simulink model "DPT_Posl_Podkl"  (R2023a)
settings: Solver=VariableStepAuto  StartTime=0.0  StopTime=10.0  RelTol=1e-3
values from neighbouring files (symbols this model uses):
  beta = 0.001    [Constants.m]
  C_m = 1.3    [Constants.m]
  C_w = 3.15    [Constants.m]
  J_dv = 7 * 10^(-6)    (= 7e-06)    [Constants.m]
  L_a = 0.0015    [Constants.m]
  L_ov = 0.013    [Constants.m]
  R_a = 8    [Constants.m]
settings Model: Creator=George  LastModifiedBy=George

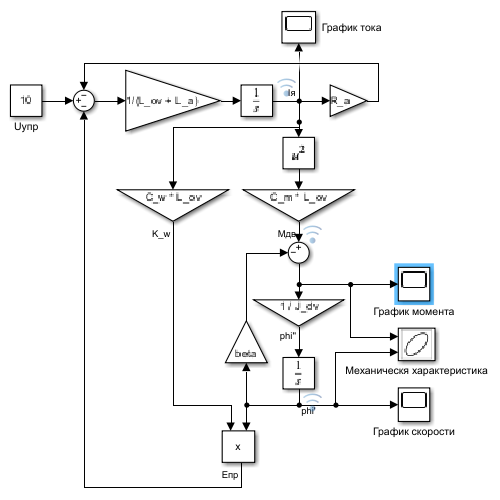
[thumbnail: Simulink's stored preview of the top-level diagram]
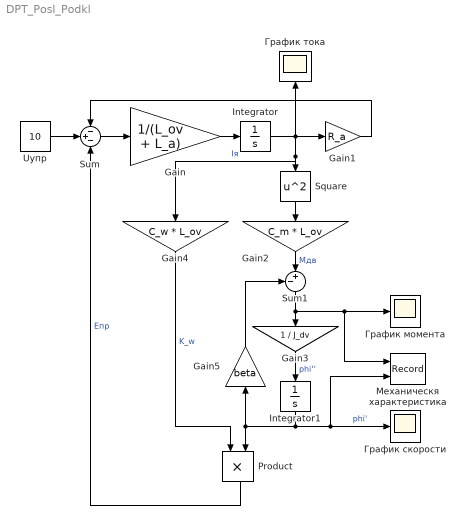
== system DPT_Posl_Podkl ==
  Gain : Gain  Gain=1/(L_ov + L_a)
  Gain1 : Gain  Gain=R_a
  Gain2 : Gain  Gain=C_m * L_ov
  Gain3 : Gain  Gain=1 / J_dv
  Gain4 : Gain  Gain=C_w * L_ov
  Gain5 : Gain  Gain=beta
  Integrator : Integrator
  Integrator1 : Integrator
  Product : Product
  Square : Math  Operator=square
  Sum : Sum  Inputs=-+-
  Sum1 : Sum  Inputs=-+|
  Uупр : Constant  Value=10
  График момента : Scope
  График скорости : Scope
  График тока : Scope
  Механическя характеристика : Record  FileSettingsInternal="{\"entries\":[{\"content\":{\"excelSettings\":{\"content\":{},\"type\":\"Streamout.ExcelSettings\"}},\"type\":\"Streamout.FileSettingStorage\",\"uuid\":\"0fa29f65-9ca5-4169-a67a-edd23fa3a2cd\"}],\"packageUris\":[\"http://schema.mathworks.com/mf0/streamout_blocks/R2020a\"],\"version\":\"1.0\"}"  Layout=[1 1]  SignalsInternal="{\"entries\":[{\"content\":{\"signals\":[{\"content\":{\"blockPath\":[\"DPT_Posl_Podkl/Механическя характеристика\"],\"dimensions\":[1],\"domain\":\"DPT_Posl_Podkl/￐ﾜ￐ﾵ￑ﾅ￐ﾰ￐ﾽ￐ﾸ￑ﾇ￐ﾵ￑ﾁ￐ﾺ￑ﾏ ￑ﾅ￐ﾰ￑ﾀ￐ﾰ￐ﾺ￑ﾂ￐ﾵ￑ﾀ￐ﾸ￑ﾁ￑ﾂ￐ﾸ￐ﾺ￐ﾰ\",\"lineColor\":\"#a2142f\",\"plots\":[1],\"port\":1,\"sid\":[\"\"],\"signalID\":202,\"signalName\":\"Sum1\"},\"type\":\"RecordBlkView.Signal\",\"uuid\":\"2999cf1a-04ad-45f2-a345-5c2da9f807c2\"},{\"content\":{\"blockPath\":[\"DPT_Posl_Podkl/Механическя характеристика\"],\"dimensions\":[1],\"domain\":\"DPT_Posl_Podkl/￐ﾜ￐ﾵ￑ﾅ￐ﾰ￐ﾽ￐ﾸ￑ﾇ￐ﾵ￑ﾁ￐ﾺ￑ﾏ ￑ﾅ￐ﾰ￑ﾀ￐ﾰ￐ﾺ￑ﾂ￐ﾵ￑ﾀ￐ﾸ￑ﾁ￑ﾂ￐ﾸ￐ﾺ￐ﾰ\",\"lineColor\":\"#139fff\",\"plots\":[1],\"port\":2,\"sid\":[\"\"],\"signalID\":206,\"signalName\":\"phi'\"},\"type\":\"RecordBlkView.Signal\",\"uuid\":\"1790a3f2-3619-4295-be67-3da603a5bf37\"}]},\"type\":\"RecordBlkView.InputSignals\",\"uuid\":\"1286b2f1-1302-4544-b370-ef9dda3b2791\"}],\"packageUris\":[\"http://schema.mathworks.com/mf0/streamout_blocks/R2020a\"],\"version\":\"1.0\"}"  VisualizationBindings="{\"xyplotplugin\":{\"info\":[{\"series\":[{\"bindingParametersList\":[{\"parameter\":\"X-Axis\",\"signalID\":202,\"signalName\":\"Sum1\"},{\"parameter\":\"Y-Axis\",\"signalID\":206,\"signalName\":\"phi'\"}],\"seriesID\":21956}],\"subplotID\":1}]}}"  CompatibilityTag=XY
  wires:
  Uупр/1 -> Sum/2
  Sum/1 -> Gain/1
  Gain/1 -> Integrator/1
  Integrator/1 -> График тока/1, Gain4/1, Square/1, Gain1/1  "Iя"
  Gain1/1 -> Sum/1
  Gain3/1 -> Integrator1/1  "phi''"
  Square/1 -> Gain2/1
  Integrator1/1 -> Gain5/1, Product/2, Механическя характеристика/2, График скорости/1  "phi'"
  Gain4/1 -> Product/1  "K_w"
  Product/1 -> Sum/3  "Eпр"
  Gain2/1 -> Sum1/2  "Mдв"
  Sum1/1 -> Механическя характеристика/1, График момента/1, Gain3/1
  Gain5/1 -> Sum1/1
